simulink model "LKAS_AutoSave_DF_20220408_1006_SW62"  (R2018b)
settings: Solver=FixedStepDiscrete  StartTime=0.0  StopTime=10.0  FixedStep=0.01  RelTol=1e-3
undefined symbols (not defined in the file): LKA_CarWidth, LKA_SampleTime, LKA_StrRatio_C, LKA_Veh2CamL_C, LKA_Veh2CamW_C, LKA_WhlBaseL_C, LL_CompHdAg_C, LL_CompSWA_C, LL_CrvtPrvwT_C, LL_DesDvt_C, LL_DvtComp_C, LL_DvtPrvwT_C, LL_DvtSpdDet_vDvtSpdMin_C, LL_HandsOff_ExitTime, LL_HandsOff_TextTime, LL_HandsOff_WarnTime, LL_HdAgExT_C, LL_HdAgPrvwT_C, LL_LAccMax_C, LL_LAccRMax_C, LL_LDW_EarliestWarnLine_C, LL_LDW_LatestWarnLine_C, LL_LDWS_SUPPRESS_HEADING, LL_LFClb_TFC_FfCtlRatio_C, LL_LFClb_TFC_KdBalance_C, LL_LFClb_TFC_KdMaxSWA_C, LL_LFClb_TFC_KdV1_C, LL_LFClb_TFC_KdV2_C, LL_LFClb_TFC_KdVehSpdLwr_C, LL_LFClb_TFC_KdVehSpdUpr_C, LL_LFClb_TFC_Ki_C, LL_LFClb_TFC_KiMaxSWA_C, LL_LFClb_TFC_Kp_C, LL_LFClb_TFC_KpKlat_C, LL_LFClb_TFC_KpV1_C, LL_LFClb_TFC_KpV2_C, LL_LFClb_TFC_KpVehSpdLwr_C, LL_LFClb_TFC_KpVehSpdUpr_C, LL_LFClb_TFC_PrvwT_C, LL_LKA_EarliestWarnLine_C, LL_LKA_LatestWarnLine_C, LL_LKAExPrcs_ExitC0Dvt, LL_LKAExPrcs_ExitC0Swt, LL_LKAExPrcs_tiExitDelayTime3, LL_LKAExPrcs_tiExitTime1, LL_LKAExPrcs_tiExitTime2, LL_LKAExPrcs_tiExitTime3, LL_LKAS_OUT_OF_CONTROL_LAT_VEL, LL_LKAS_OUT_OF_CONTROL_TTLC, LL_LKASWASyn_M0, LL_LKASWASyn_M1, LL_LKASWASyn_M2, LL_LKASWASyn_M3D, LL_LKASWASyn_M3K_DT, LL_LKASWASyn_M3K_MSD, LL_LKASWASyn_M4K, LL_LKASWASyn_SWAaddMax, LL_LKASWASyn_T2, LL_LKASWASyn_tiTrqSwaRtTime, LL_LKASWASyn_tiTrqSwaTime ... (+47)
libraries: simulink x234, canmsglib x6, dspstat3 x3, simulink_extras x1
(part 3 of 16)

== system LKAS_AutoSave_DF_20220408_1006_SW62/LKAS/Output ==
  bsLLOut : Inport
  Bus Selector : BusSelector  OutputSignals=Vehicle_Lane_Display,LDW_Status_Display,LKA_Status_Display,LDW_Flag,Hands_Off_Warning,HapticAlarmReq,LKA_Action_Indication,HMI_Popup_Status,LKA_Torque_Req,LKA_TorqueReq_Value,EPS_State_Ctl,LKA_SWA_Control,EPS_Factor_Control,EPS_LKA_Control
  Cast To Single{1..9,12,14..16} (13 alike) : DataTypeConversion  OutDataTypeStr=UInt8
  Cast To Single10 : DataTypeConversion  OutDataTypeStr=T_M_Nm_Float32
  Cast To Single11 : DataTypeConversion  OutDataTypeStr=T_M_Nm_Float32
  Cast To Single13 : DataTypeConversion  OutDataTypeStr=T_M_Nm_Float32
  Ground : Ground
  Ground1 : Ground
  Vehicle_Lane_Display : Outport
  LDW_Status_Display : Outport  Port=2
  LKA_Status_Display : Outport  Port=3
  ELK_Status_Display : Outport  Port=4
  LDW_Flag : Outport  Port=5
  Hands_Off_Warning : Outport  Port=6
  HapticAlarmReq : Outport  Port=7
  LKA_Action_Indication : Outport  Port=8
  HMI_Popup_Status : Outport  Port=9
  HMI_ELKPopupMessage : Outport  Port=10
  LKA_TorqueReq : Outport  Port=11
  LKA_TorqueReq_Value : Outport  Port=12
  EPS_State_Control : Outport  Port=13
  LKA_SWA_Control : Outport  Port=14
  EPS_Factor_Control : Outport  Port=15
  EPS_LKA_Control : Outport  Port=16
  wires:
  Ground1/1 -> Cast To Single16/1  "<HMI_ELKPopupMessage>"
  Bus Selector/6 -> Cast To Single15/1  "<HapticAlarmReq>"
  Ground/1 -> Cast To Single14/1  "<ELK_Status_Display>"
  Cast To Single16/1 -> HMI_ELKPopupMessage/1  "HMI_ELKPopupMessage"
  Cast To Single14/1 -> ELK_Status_Display/1  "ELK_Status_Display"
  Cast To Single15/1 -> HapticAlarmReq/1  "HapticAlarmReq"
  Bus Selector/2 -> Cast To Single2/1  "<LDW_Status_Display>"
  Bus Selector/14 -> Cast To Single9/1  "<EPS_LKA_Control>"
  Bus Selector/12 -> Cast To Single11/1  "<LKA_SWA_Control>"
  bsLLOut/1 -> Bus Selector/1  "bsLLOutput"
  Bus Selector/11 -> Cast To Single8/1  "<EPS_State_Ctl>"
  Bus Selector/1 -> Cast To Single1/1  "<Vehicle_Lane_Display>"
  Bus Selector/5 -> Cast To Single5/1  "<Hands_Off_Warning>"
  Bus Selector/8 -> Cast To Single7/1  "<HMI_Popup_Status>"
  Bus Selector/7 -> Cast To Single6/1  "<LKA_Action_Indication>"
  Bus Selector/13 -> Cast To Single10/1  "<EPS_Factor_Control>"
  Bus Selector/3 -> Cast To Single3/1  "<LKA_Status_Display>"
  Bus Selector/4 -> Cast To Single4/1  "<LDW_Flag>"
  Bus Selector/9 -> Cast To Single12/1  "<LKA_Torque_Req>"
  Bus Selector/10 -> Cast To Single13/1  "<LKA_TorqueReq_Value>"
  Cast To Single13/1 -> LKA_TorqueReq_Value/1  "LKA_TorqueReq_Value"
  Cast To Single12/1 -> LKA_TorqueReq/1  "LKA_TorqueReq"
  Cast To Single11/1 -> LKA_SWA_Control/1  "LKA_SWA_Control"
  Cast To Single10/1 -> EPS_Factor_Control/1  "EPS_Factor_Control"
  Cast To Single9/1 -> EPS_LKA_Control/1  "EPS_LKA_Control"
  Cast To Single8/1 -> EPS_State_Control/1  "EPS_State_Control"
  Cast To Single7/1 -> HMI_Popup_Status/1  "HMI_Popup_Status"
  Cast To Single6/1 -> LKA_Action_Indication/1  "LKA_Action_Indication"
  Cast To Single5/1 -> Hands_Off_Warning/1  "Hands_Off_Warning"
  Cast To Single4/1 -> LDW_Flag/1  "LDW_Flag"
  Cast To Single3/1 -> LKA_Status_Display/1  "LKA_Status_Display"
  Cast To Single2/1 -> LDW_Status_Display/1  "LDW_Status_Display"
  Cast To Single1/1 -> Vehicle_Lane_Display/1  "Vehicle_Lane_Display"

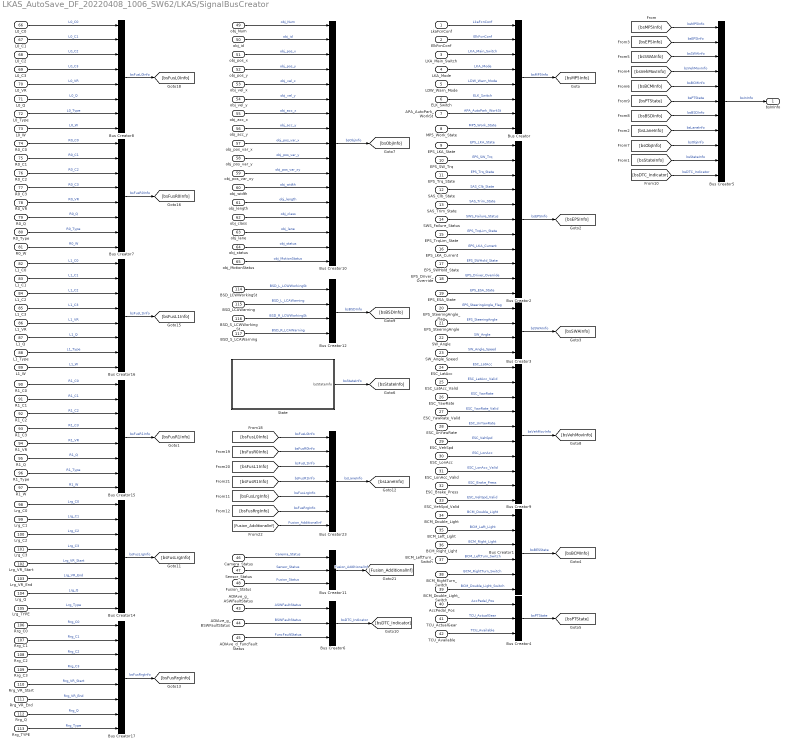
== system LKAS_AutoSave_DF_20220408_1006_SW62/LKAS/SignalBusCreator ==
  LkaFcnConf : Inport
  ElkFcnConf : Inport  Port=2
  LKA_Main_Switch : Inport  Port=3
  LKA_Mode : Inport  Port=4
  LDW_Warn_Mode : Inport  Port=5
  ELK_Switch : Inport  Port=6
  APA_AutoPark_WorkSt : Inport  Port=7
  MP5_Work_State : Inport  Port=8
  EPS_LKA_State : Inport  Port=9
  EPS_SW_Trq : Inport  Port=10
  EPS_Trq_State : Inport  Port=11
  SAS_Clb_State : Inport  Port=12
  SAS_Trim_State : Inport  Port=13
  SWS_Failure_Status : Inport  Port=14
  EPS_TrqLim_State : Inport  Port=15
  EPS_LKA_Current : Inport  Port=16
  EPS_SWHold_State : Inport  Port=17
  EPS_Driver_Override : Inport  Port=18
  EPS_ESA_State : Inport  Port=19
  EPS_SteeringAngle_Flag : Inport  Port=20
  EPS_SteeringAngle : Inport  Port=21
  SW_Angle : Inport  Port=22
  SW_Angle_Speed : Inport  Port=23
  ESC_LatAcc : Inport  Port=24
  ESC_LatAcc_Valid : Inport  Port=25
  ESC_YawRate : Inport  Port=26
  ESC_YawRate_Valid : Inport  Port=27
  ESC_UnYawRate : Inport  Port=28
  ESC_VehSpd : Inport  Port=29
  ESC_LonAcc : Inport  Port=30
  ESC_LonAcc_Valid : Inport  Port=31
  ESC_Brake_Press : Inport  Port=32
  ESC_VehSpd_Valid : Inport  Port=33
  BCM_Double_Light : Inport  Port=34
  BCM_Left_Light : Inport  Port=35
  BCM_Right_Light : Inport  Port=36
  BCM_LeftTurn_Switch : Inport  Port=37
  BCM_RightTurn_Switch : Inport  Port=38
  BCM_Double_Light_Switch : Inport  Port=39
  AccPedal_Pos : Inport  Port=40
  TCU_ActualGear : Inport  Port=41
  TCU_Available : Inport  Port=42
  ADIAve_g_ASWFaultStatus : Inport  Port=43
  ADIAve_g_BSWFaultStatus : Inport  Port=44
  ADIAve_d_FuncFaultStatus : Inport  Port=45
  Camera_Status : Inport  Port=46
  Sensor_Status : Inport  Port=47
  Fusion_Status : Inport  Port=48
  obj_Num : Inport  Port=49
  obj_id : Inport  Port=50
  obj_pos_x : Inport  Port=51
  obj_pos_y : Inport  Port=52
  obj_vel_x : Inport  Port=53
  obj_vel_y : Inport  Port=54
  obj_acc_x : Inport  Port=55
  obj_acc_y : Inport  Port=56
  obj_pos_var_x : Inport  Port=57
  obj_pos_var_y : Inport  Port=58
  obj_pos_var_xy : Inport  Port=59
  obj_width : Inport  Port=60
  obj_length : Inport  Port=61
  obj_class : Inport  Port=62
  obj_lane : Inport  Port=63
  obj_status : Inport  Port=64
  obj_MotionStatus : Inport  Port=65
  L0_C0 : Inport  Port=66
  L0_C1 : Inport  Port=67
  L0_C2 : Inport  Port=68
  L0_C3 : Inport  Port=69
  L0_VR : Inport  Port=70
  L0_Q : Inport  Port=71
  L0_Type : Inport  Port=72
  L0_W : Inport  Port=73
  R0_C0 : Inport  Port=74
  R0_C1 : Inport  Port=75
  R0_C2 : Inport  Port=76
  R0_C3 : Inport  Port=77
  R0_VR : Inport  Port=78
  R0_Q : Inport  Port=79
  R0_Type : Inport  Port=80
  R0_W : Inport  Port=81
  L1_C0 : Inport  Port=82
  L1_C1 : Inport  Port=83
  L1_C2 : Inport  Port=84
  L1_C3 : Inport  Port=85
  L1_VR : Inport  Port=86
  L1_Q : Inport  Port=87
  L1_Type : Inport  Port=88
  L1_W : Inport  Port=89
  R1_C0 : Inport  Port=90
  R1_C1 : Inport  Port=91
  R1_C2 : Inport  Port=92
  R1_C3 : Inport  Port=93
  R1_VR : Inport  Port=94
  R1_Q : Inport  Port=95
  R1_Type : Inport  Port=96
  R1_W : Inport  Port=97
  Lrg_C0 : Inport  Port=98
  Lrg_C1 : Inport  Port=99
  Lrg_C2 : Inport  Port=100
  Lrg_C3 : Inport  Port=101
  Lrg_VR_Start : Inport  Port=102
  Lrg_VR_End : Inport  Port=103
  Lrg_Q : Inport  Port=104
  Lrg_TYPE : Inport  Port=105
  Rrg_C0 : Inport  Port=106
  Rrg_C1 : Inport  Port=107
  Rrg_C2 : Inport  Port=108
  Rrg_C3 : Inport  Port=109
  Rrg_VR_Start : Inport  Port=110
  Rrg_VR_End : Inport  Port=111
  Rrg_Q : Inport  Port=112
  Rrg_TYPE : Inport  Port=113
  BSD_LCWWorkingSt : Inport  Port=114
  BSD_LCAWarning : Inport  Port=115
  BSD_S_LCWWorkingSt : Inport  Port=116
  BSD_S_LCAWarning : Inport  Port=117
  Bus Creator{,7..8,14..17} (7 alike) : BusCreator  Inputs=8
  Bus Creator1 : BusCreator  Inputs=6
  Bus Creator10 : BusCreator  Inputs=17
  Bus Creator11 : BusCreator  Inputs=3
  Bus Creator12 : BusCreator  Inputs=4
  Bus Creator2 : BusCreator  Inputs=11
  Bus Creator23 : BusCreator  Inputs=7
  Bus Creator3 : BusCreator  Inputs=4
  Bus Creator4 : BusCreator  Inputs=3
  Bus Creator5 : BusCreator  Inputs=11
  Bus Creator6 : BusCreator  Inputs=3
  Bus Creator9 : BusCreator  Inputs=10
  State : Subsystem
  bsInInfo : Outport
  wires:
  [bsFusRrgInfo] -> Bus Creator23/6  "bsFusRrgInfo"
  [bsFusLrgInfo] -> Bus Creator23/5  "bsFusLrgInfo"
  Rrg_TYPE/1 -> Bus Creator17/8  "Rrg_Type"
  Rrg_Q/1 -> Bus Creator17/7  "Rrg_Q"
  Rrg_VR_End/1 -> Bus Creator17/6  "Rrg_VR_End"
  Rrg_VR_Start/1 -> Bus Creator17/5  "Rrg_VR_Start"
  Rrg_C3/1 -> Bus Creator17/4  "Rrg_C3"
  Rrg_C2/1 -> Bus Creator17/3  "Rrg_C2"
  Rrg_C1/1 -> Bus Creator17/2  "Rrg_C1"
  Rrg_C0/1 -> Bus Creator17/1  "Rrg_C0"
  Bus Creator17/1 -> [bsFusRrgInfo]  "bsFusRrgInfo"
  Bus Creator14/1 -> [bsFusLrgInfo]  "bsFusLrgInfo"
  Lrg_TYPE/1 -> Bus Creator14/8  "Lrg_Type"
  Lrg_Q/1 -> Bus Creator14/7  "Lrg_Q"
  Lrg_VR_End/1 -> Bus Creator14/6  "Lrg_VR_End"
  Lrg_VR_Start/1 -> Bus Creator14/5  "Lrg_VR_Start"
  Lrg_C3/1 -> Bus Creator14/4  "Lrg_C3"
  Lrg_C2/1 -> Bus Creator14/3  "Lrg_C2"
  Lrg_C1/1 -> Bus Creator14/2  "Lrg_C1"
  Lrg_C0/1 -> Bus Creator14/1  "Lrg_C0"
  [bsBSDInfo] -> Bus Creator5/7  "bsBSDInfo"
  Bus Creator12/1 -> [bsBSDInfo]  "bsBSDInfo"
  BSD_S_LCAWarning/1 -> Bus Creator12/4  "BSD_R_LCAWarning"
  BSD_S_LCWWorkingSt/1 -> Bus Creator12/3  "BSD_R_LCWWorkingSt"
  BSD_LCAWarning/1 -> Bus Creator12/2  "BSD_L_LCAWarning"
  BSD_LCWWorkingSt/1 -> Bus Creator12/1  "BSD_L_LCWWorkingSt"
  [bsObjInfo] -> Bus Creator5/9  "bsObjInfo"
  Bus Creator10/1 -> [bsObjInfo]  "bsObjInfo"
  obj_MotionStatus/1 -> Bus Creator10/17  "obj_MotionStatus"
  obj_status/1 -> Bus Creator10/16  "obj_status"
  obj_lane/1 -> Bus Creator10/15  "obj_lane"
  obj_class/1 -> Bus Creator10/14  "obj_class"
  obj_length/1 -> Bus Creator10/13  "obj_length"
  obj_width/1 -> Bus Creator10/12  "obj_width"
  obj_pos_var_xy/1 -> Bus Creator10/11  "obj_pos_var_xy"
  obj_pos_var_y/1 -> Bus Creator10/10  "obj_pos_var_y"
  obj_pos_var_x/1 -> Bus Creator10/9  "obj_pos_var_x"
  obj_acc_y/1 -> Bus Creator10/8  "obj_acc_y"
  obj_acc_x/1 -> Bus Creator10/7  "obj_acc_x"
  obj_vel_y/1 -> Bus Creator10/6  "obj_vel_y"
  obj_vel_x/1 -> Bus Creator10/5  "obj_vel_x"
  obj_pos_y/1 -> Bus Creator10/4  "obj_pos_y"
  obj_pos_x/1 -> Bus Creator10/3  "obj_pos_x"
  obj_id/1 -> Bus Creator10/2  "obj_id"
  obj_Num/1 -> Bus Creator10/1  "obj_Num"
  ELK_Switch/1 -> Bus Creator/6  "ELK_Switch"
  ElkFcnConf/1 -> Bus Creator/2  "ElkFcnConf"
  BCM_Double_Light_Switch/1 -> Bus Creator1/6  "BCM_Double_Light_Switch"
  ADIAve_d_FuncFaultStatus/1 -> Bus Creator6/3  "FuncFaultStatus"
  ADIAve_g_BSWFaultStatus/1 -> Bus Creator6/2  "BSWFaultStatus"
  ADIAve_g_ASWFaultStatus/1 -> Bus Creator6/1  "ASWFaultStatus"
  EPS_ESA_State/1 -> Bus Creator2/11  "EPS_ESA_State"
  LkaFcnConf/1 -> Bus Creator/1  "LkaFcnConf"
  LDW_Warn_Mode/1 -> Bus Creator/5  "LDW_Warn_Mode"
  APA_AutoPark_WorkSt/1 -> Bus Creator/7  "APA_AutoPark_WorkSt"
  MP5_Work_State/1 -> Bus Creator/8  "MP5_Work_State"
  Fusion_Status/1 -> Bus Creator11/3  "Fusion_Status"
  Sensor_Status/1 -> Bus Creator11/2  "Sensor_Status"
  Camera_Status/1 -> Bus Creator11/1  "Carema_Status"
  Bus Creator11/1 -> [Fusion_AdditionalInf]  "Fusion_AdditionalInf"
  EPS_Driver_Override/1 -> Bus Creator2/10  "EPS_Driver_Override"
  EPS_SteeringAngle/1 -> Bus Creator3/2  "EPS_SteeringAngle"
  EPS_SteeringAngle_Flag/1 -> Bus Creator3/1  "EPS_SteeringAngle_Flag"
  BCM_RightTurn_Switch/1 -> Bus Creator1/5  "BCM_RightTurn_Switch"
  BCM_LeftTurn_Switch/1 -> Bus Creator1/4  "BCM_LeftTurn_Switch"
  TCU_Available/1 -> Bus Creator4/3  "TCU_Available"
  R1_W/1 -> Bus Creator15/8  "R1_W"
  R1_Type/1 -> Bus Creator15/7  "R1_Type"
  R1_Q/1 -> Bus Creator15/6  "R1_Q"
  R1_VR/1 -> Bus Creator15/5  "R1_VR"
  R1_C3/1 -> Bus Creator15/4  "R1_C3"
  R1_C2/1 -> Bus Creator15/3  "R1_C2"
  R1_C1/1 -> Bus Creator15/2  "R1_C1"
  R1_C0/1 -> Bus Creator15/1  "R1_C0"
  L1_W/1 -> Bus Creator16/8  "L1_W"
  L1_Type/1 -> Bus Creator16/7  "L1_Type"
  L1_Q/1 -> Bus Creator16/6  "L1_Q"
  L1_VR/1 -> Bus Creator16/5  "L1_VR"
  L1_C3/1 -> Bus Creator16/4  "L1_C3"
  L1_C2/1 -> Bus Creator16/3  "L1_C2"
  L1_C1/1 -> Bus Creator16/2  "L1_C1"
  L1_C0/1 -> Bus Creator16/1  "L1_C0"
  R0_W/1 -> Bus Creator7/8  "R0_W"
  R0_Type/1 -> Bus Creator7/7  "R0_Type"
  R0_Q/1 -> Bus Creator7/6  "R0_Q"
  R0_VR/1 -> Bus Creator7/5  "R0_VR"
  R0_C3/1 -> Bus Creator7/4  "R0_C3"
  R0_C2/1 -> Bus Creator7/3  "R0_C2"
  R0_C1/1 -> Bus Creator7/2  "R0_C1"
  R0_C0/1 -> Bus Creator7/1  "R0_C0"
  L0_W/1 -> Bus Creator8/8  "L0_W"
  L0_Type/1 -> Bus Creator8/7  "L0_Type"
  L0_Q/1 -> Bus Creator8/6  "L0_Q"
  L0_VR/1 -> Bus Creator8/5  "L0_VR"
  L0_C3/1 -> Bus Creator8/4  "L0_C3"
  L0_C2/1 -> Bus Creator8/3  "L0_C2"
  L0_C1/1 -> Bus Creator8/2  "L0_C1"
  L0_C0/1 -> Bus Creator8/1  "L0_C0"
  LKA_Mode/1 -> Bus Creator/4  "LKA_Mode"
  LKA_Main_Switch/1 -> Bus Creator/3  "LKA_Main_Switch"
  EPS_SWHold_State/1 -> Bus Creator2/9  "EPS_SWHold_State"
  EPS_LKA_Current/1 -> Bus Creator2/8  "EPS_LKA_Current"
  EPS_TrqLim_State/1 -> Bus Creator2/7  "EPS_TrqLim_State"
  SAS_Trim_State/1 -> Bus Creator2/5  "SAS_Trim_State"
  SAS_Clb_State/1 -> Bus Creator2/4  "SAS_Clb_State"
  EPS_Trq_State/1 -> Bus Creator2/3  "EPS_Trq_State"
  EPS_SW_Trq/1 -> Bus Creator2/2  "EPS_SW_Trq"
  EPS_LKA_State/1 -> Bus Creator2/1  "EPS_LKA_State"
  ESC_VehSpd_Valid/1 -> Bus Creator9/10  "ESC_VehSpd_Valid"
  ESC_Brake_Press/1 -> Bus Creator9/9  "ESC_Brake_Press"
  ESC_LonAcc_Valid/1 -> Bus Creator9/8  "ESC_LonAcc_Valid"
  ESC_LonAcc/1 -> Bus Creator9/7  "ESC_LonAcc"
  ESC_VehSpd/1 -> Bus Creator9/6  "ESC_VehSpd"
  ESC_UnYawRate/1 -> Bus Creator9/5  "ESC_UnYawRate"
  ESC_YawRate_Valid/1 -> Bus Creator9/4  "ESC_YawRate_Valid"
  ESC_YawRate/1 -> Bus Creator9/3  "ESC_YawRate"
  ESC_LatAcc_Valid/1 -> Bus Creator9/2  "ESC_LatAcc_Valid"
  ESC_LatAcc/1 -> Bus Creator9/1  "ESC_LatAcc"
  SWS_Failure_Status/1 -> Bus Creator2/6  "SWS_Failure_Status"
  SW_Angle_Speed/1 -> Bus Creator3/4  "SW_Angle_Speed"
  SW_Angle/1 -> Bus Creator3/3  "SW_Angle"
  BCM_Right_Light/1 -> Bus Creator1/3  "BCM_Right_Light"
  BCM_Left_Light/1 -> Bus Creator1/2  "BCM_Left_Light"
  BCM_Double_Light/1 -> Bus Creator1/1  "BCM_Double_Light"
  TCU_ActualGear/1 -> Bus Creator4/2  "TCU_ActualGear"
  AccPedal_Pos/1 -> Bus Creator4/1  "AccPedal_Pos"
  Bus Creator5/1 -> bsInInfo/1  "bsInInfo"
  State/1(bsStateInfo) -> [bsStateInfo]  "bsStateInfo"
  Bus Creator6/1 -> [bsDTC_Indicator]  "bsDTC_Indicator"
  [Fusion_AdditionalInf] -> Bus Creator23/7  "Fusion_AdditionalInf"
  Bus Creator23/1 -> [bsLaneInfo]  "bsLaneInfo"
  [bsFusR1Info] -> Bus Creator23/4  "bsFusR1Info"
  [bsFusL1Info] -> Bus Creator23/3  "bsFusL1Info"
  [bsFusR0Info] -> Bus Creator23/2  "bsFusR0Info"
  [bsFusL0Info] -> Bus Creator23/1  "bsFusL0Info"
  Bus Creator8/1 -> [bsFusL0Info]  "bsFusL0Info"
  Bus Creator15/1 -> [bsFusR1Info]  "bsFusR1Info"
  Bus Creator16/1 -> [bsFusL1Info]  "bsFusL1Info"
  Bus Creator7/1 -> [bsFusR0Info]  "bsFusR0Info"
  Bus Creator4/1 -> [bsPTState]  "bsPTState"
  [bsDTC_Indicator] -> Bus Creator5/11  "bsDTC_Indicator"
  [bsStateInfo] -> Bus Creator5/10  "bsStateInfo"
  [bsMP5Info] -> Bus Creator5/1  "bsMP5Info"
  [bsPTState] -> Bus Creator5/6  "bsPTState"
  [bsBCMInfo] -> Bus Creator5/5  "bsBCMInfo"
  [bsSWAInfo] -> Bus Creator5/3  "bsSWAInfo"
  [bsVehMovInfo] -> Bus Creator5/4  "bsVehMovInfo"
  [bsEPSInfo] -> Bus Creator5/2  "bsEPSInfo"
  [bsLaneInfo] -> Bus Creator5/8  "bsLaneInfo"
  Bus Creator/1 -> [bsMP5Info]  "bsMP5Info"
  Bus Creator2/1 -> [bsEPSInfo]  "bsEPSInfo"
  Bus Creator1/1 -> [bsBCMInfo]  "bsBESState"
  Bus Creator3/1 -> [bsSWAInfo]  "bsSWAInfo"
  Bus Creator9/1 -> [bsVehMovInfo]  "bsVehMovInfo"

== system LKAS_AutoSave_DF_20220408_1006_SW62/LKAS/LL/Fault_Diagnostic ==
  bsInInfo : Inport
  ASWFaultStatus_Unpack : Subsystem
  BSWFaultStatus_Unpack : Subsystem
  Bus Creator : BusCreator  Inputs=3
  Bus Selector4 : BusSelector  OutputSignals=bsDTC_Indicator.ASWFaultStatus,bsDTC_Indicator.BSWFaultStatus,bsDTC_Indicator.FuncFaultStatus
  FuncFaultStatus_Unpack : Subsystem
  bsFaultStatus : Outport
  wires:
  Bus Creator/1 -> bsFaultStatus/1  "bsFaultStatus"
  FuncFaultStatus_Unpack/1(bsFuncFaultStatus) -> Bus Creator/3  "bsFuncFaultStatus"
  BSWFaultStatus_Unpack/1(bsBSWFaultStatus) -> Bus Creator/2  "bsBSWFaultStatus"
  ASWFaultStatus_Unpack/1(bsASWFaultStatus) -> Bus Creator/1  "bsASWFaultStatus"
  [FuncFaultStatus] -> FuncFaultStatus_Unpack/1(FuncFaultStatus)
  [BSWFaultStatus] -> BSWFaultStatus_Unpack/1(BSWFaultStatus), ASWFaultStatus_Unpack/2(BSWFaultStatus)
  [ASWFaultStatus] -> ASWFaultStatus_Unpack/1(ASWFaultStatus)
  Bus Selector4/3 -> [FuncFaultStatus]  "<FuncFaultStatus>"
  Bus Selector4/2 -> [BSWFaultStatus]  "<BSWFaultStatus>"
  Bus Selector4/1 -> [ASWFaultStatus]  "<ASWFaultStatus>"
  bsInInfo/1 -> Bus Selector4/1

== system LKAS_AutoSave_DF_20220408_1006_SW62/LKAS/LL/Human Machine Interface (HMI) ==
  HMI_bsInfo : Inport
  HMI_bsLLState : Inport  Port=2
  HMI_bsLDWWarnInfo : Inport  Port=3
  HMI_bsLLClb : Inport  Port=4
  Bus Creator2 : BusCreator  Inputs=8
  Bus Selector : BusSelector  OutputSignals=bsConstantClb.LKA_SampleTime,bsLLSMConClb.DisblCClb.LL_HandsOff_TextTime,bsLLSMConClb.DisblCClb.LL_HandsOff_WarnTime,bsLLSMConClb.DisblCClb.LL_RlsDet_tiTrqChkT_DISABLE,bsLLSMConClb.DisblCClb.LL_RlsDet_tiTrqChkT_EPS_DISABLE
  Bus Selector1 : BusSelector  OutputSignals=LKA_Mode,LKA_State,LDW_State
  Bus Selector5 : BusSelector  OutputSignals=bsLaneInfo.bsR0Info.R0_Q,bsLaneInfo.bsL0Info.L0_Q,bsLaneInfo.Fusion_AdditionalInf.Carema_Status,bsEPSInfo,bsMP5Info.LDW_Warn_Mode
  Cast To Single{,1..6,8} (8 alike) : DataTypeConversion  OutDataTypeStr=uint8
  HMI_Popup_Status : MATLAB Function  TreatAsAtomicUnit=on
  Hands_Off_Warning : MATLAB Function  TreatAsAtomicUnit=on
  HapticAlarmReq : MATLAB Function  TreatAsAtomicUnit=on
  LDW_Flag : MATLAB Function  TreatAsAtomicUnit=on
  LKA_action_indication : MATLAB Function  TreatAsAtomicUnit=on
  Status_Display : MATLAB Function  TreatAsAtomicUnit=on
  Subsystem : Subsystem
  Vehicle_Lane_Display : MATLAB Function  TreatAsAtomicUnit=on
  HMI_LDWLKA : Outport
  wires:
  Bus Selector/5 -> Subsystem/8(LL_RlsDet_tiTrqChkT_EPS_DISABLE)  "<LL_RlsDet_tiTrqChkT_EPS_DISABLE>"
  Bus Selector/4 -> Subsystem/7(LL_RlsDet_tiTrqChkT_DISABLE)  "<LL_RlsDet_tiTrqChkT_DISABLE>"
  [HMI_Popup_Status] -> Cast To Single6/1
  [LKA_Action_Indication] -> Cast To Single5/1
  [HapticAlarmReq] -> Cast To Single8/1
  [LDW_Flag] -> HapticAlarmReq/2(LDW_Flag)
  Bus Selector5/5 -> LDW_Flag/4(LDW_Warn_Mode), HapticAlarmReq/1(LDW_Warn_Mode)  "<LDW_Warn_Mode>"
  [LDW_Flag] -> Cast To Single3/1
  [Hands_Off_Warning] -> Cast To Single4/1
  [LKA_Status_Display] -> Cast To Single2/1
  [LDW_Status_Display] -> Cast To Single1/1
  [Vehicle_Lane_Display] -> Cast To Single/1
  HMI_bsLLState/1 -> Bus Selector1/1
  HMI_bsInfo/1 -> Bus Selector5/1
  HapticAlarmReq/1(HapticAlarmReq) -> [HapticAlarmReq]  "HapticAlarmReq"
  Cast To Single8/1 -> Bus Creator2/6  "HapticAlarmReq"
  Bus Selector/3 -> Subsystem/6(LL_HandsOff_WarnTime)  "<LL_HandsOff_WarnTime>"
  Bus Selector/2 -> Subsystem/5(LL_HandsOff_TextTime)  "<LL_HandsOff_TextTime>"
  Bus Selector/1 -> Subsystem/4(LKA_SampleTime)  "<LKA_SampleTime>"
  HMI_bsLLClb/1 -> Bus Selector/1  "HMI_bsLLClb"
  HMI_bsLDWWarnInfo/1 -> LDW_Flag/3(LDWWarnInfo)
  Subsystem/1(HandsOff2_Warn) -> Hands_Off_Warning/1(HandsOff)
  Subsystem/2(HandsOff1_Text) -> HMI_Popup_Status/2(HandsOff1_Text)
  Bus Selector5/4 -> Subsystem/3(bsEPSInfo)  "<bsEPSInfo>"
  Bus Selector5/1 -> Vehicle_Lane_Display/4(R0_Q)  "<R0_Q>"
  Bus Selector5/3 -> HMI_Popup_Status/3(Camera_Status)  "<Carema_Status>"
  Bus Selector1/1 -> LDW_Flag/1(LKA_Mode), Status_Display/1(LKA_Mode), Vehicle_Lane_Display/1(LKA_Mode), LKA_action_indication/1(LKA_Mode), HMI_Popup_Status/1(LKA_Mode)  "<LKA_Mode>"
  Bus Selector5/2 -> Vehicle_Lane_Display/5(L0_Q)  "<L0_Q>"
  Bus Selector1/3 -> Subsystem/1(LDW_State), Vehicle_Lane_Display/3(LDW_State), Status_Display/2(LDW_STATE)  "<LDW_State>"
  Bus Selector1/2 -> Vehicle_Lane_Display/2(LKA_State), Status_Display/3(LKA_STATE), LDW_Flag/2(LKA_State), LKA_action_indication/2(LKA_STATE), Subsystem/2(LKA_State)  "<LKA_State>"
  Cast To Single4/1 -> Bus Creator2/5  "Hands_Off_Warning"
  LKA_action_indication/1(LKA_Action_Indication) -> [LKA_Action_Indication]  "LKA_Action_Indication"
  Cast To Single6/1 -> Bus Creator2/8  "HMI_Popup_Status"
  Cast To Single/1 -> Bus Creator2/1  "Vehicle_Lane_Display"
  Vehicle_Lane_Display/1(Vehicle_Lane_Display) -> [Vehicle_Lane_Display]  "Vehicle_Lane_Display"
  Cast To Single3/1 -> Bus Creator2/4  "LDW_Flag"
  Status_Display/2(LKA_Status_Display) -> [LKA_Status_Display]  "LKA_Status_Display"
  Cast To Single1/1 -> Bus Creator2/2  "LDW_Status_Display"
  HMI_Popup_Status/1(HMI_Popup_Status) -> [HMI_Popup_Status]  "HMI_Popup_Status"
  Status_Display/1(LDW_Status_Display) -> [LDW_Status_Display]  "LDW_Status_Display"
  LDW_Flag/1(LDW_Flag) -> [LDW_Flag]  "LDW_Flag"
  Cast To Single2/1 -> Bus Creator2/3  "LKA_Status_Display"
  Cast To Single5/1 -> Bus Creator2/7  "LKA_Action_Indication"
  Hands_Off_Warning/1(Hands_Off_Warning) -> [Hands_Off_Warning]  "Hands_Off_Warning"
  Bus Creator2/1 -> HMI_LDWLKA/1

== system LKAS_AutoSave_DF_20220408_1006_SW62/LKAS/LL/LL Inputs Mapping ==
  bsInInfo : Inport
  bsLLClb : Inport  Port=2
  Bus Creator : BusCreator  Inputs=7
  Bus Selector : BusSelector  OutputSignals=bsMP5Info,bsLaneInfo,bsEPSInfo,bsVehMovInfo,bsSWAInfo,bsBCMInfo,bsPTState
  bsBCMInfo : Subsystem
  bsEPSInfo : Subsystem
  bsLaneInfo : Subsystem
  bsMP5Info : Subsystem
  bsPTState : Subsystem
  bsSWAInfo : Subsystem
  bsVehMovInfo : Subsystem
  bsInfo : Outport
  wires:
  bsLLClb/1 -> bsLaneInfo/1(bsLLClb)
  bsInInfo/1 -> Bus Selector/1
  Bus Creator/1 -> bsInfo/1
  Bus Selector/2 -> bsLaneInfo/2(bsLaneInfoIn)  "<bsLaneInfo>"
  Bus Selector/3 -> bsEPSInfo/1(bsEPSInfoIn)  "<bsEPSInfo>"
  bsEPSInfo/1(bsEPSInfoOut) -> Bus Creator/3  "bsEPSInfo"
  Bus Selector/4 -> bsVehMovInfo/1(bsVehMovInfoIn)  "<bsVehMovInfo>"
  bsVehMovInfo/1(bsVehMovInfoOut) -> Bus Creator/4  "bsVehMovInfo"
  Bus Selector/5 -> bsSWAInfo/1(bsSWAInfoIn)  "<bsSWAInfo>"
  Bus Selector/6 -> bsBCMInfo/1(bsBCMInfoIn)  "<bsBCMInfo>"
  Bus Selector/1 -> bsMP5Info/1(bsMP5InfoIn)  "<bsMP5Info>"
  bsMP5Info/1(bsMP5InfoOut) -> Bus Creator/1  "bsMP5Info"
  bsBCMInfo/1(bsBCMInfoOut) -> Bus Creator/6  "bsBCMInfo"
  Bus Selector/7 -> bsPTState/1(bsPTStateIn)  "<bsPTState>"
  bsPTState/1(bsPTStateOut) -> Bus Creator/7  "bsPTState"
  bsLaneInfo/1(bsLaneInfoOut) -> Bus Creator/2  "bsLaneInfo"
  bsSWAInfo/1(bsSWAInfoOut) -> Bus Creator/5  "bsSWAInfo"

== system LKAS_AutoSave_DF_20220408_1006_SW62/LKAS/LL/LLOn ==
  bsInInfo : Inport
  bsLLClb : Inport  Port=2
  bsSignalFault : Inport  Port=3
  Enable : EnablePort  StatesWhenEnabling=reset
      settings: AttributesFormatString=states = %<StatesWhenEnabling>
  LDW : Subsystem  Description=|  TreatAsAtomicUnit=on
      | Block Name: Lane Departure Warning
      | Ab.: LDW
      | No.: 1.3.0.0
      | Rev: 0.0.1
      | Update Date: 19-3-26
  LKA : Subsystem  Description=|  TreatAsAtomicUnit=on
      | Block Name: Lane Keeping Assistance
      | Ab.: LKA
      | No.: 1.2.0.0
      | Rev: 0.0.1
      | Update Date: 19-5-13
  LKA Input Processing (LKAInP) : Subsystem
  LL State Determination (LLStateDet) : Subsystem
  LL_Mon : Subsystem
  bsLLState : Outport  OutputWhenDisabled=reset  InitialOutput=0
      settings: AttributesFormatString=%<OutputWhenDisabled> = %<InitialOutput>
  LDW_Flag : Outport  Port=2  OutputWhenDisabled=reset  InitialOutput=0
      settings: AttributesFormatString=%<OutputWhenDisabled> = %<InitialOutput>
  phiSWACmd : Outport  Port=3  OutputWhenDisabled=reset  InitialOutput=0
      settings: AttributesFormatString=%<OutputWhenDisabled> = %<InitialOutput>
  M : Outport  Port=4  OutputWhenDisabled=reset  InitialOutput=0
      settings: AttributesFormatString=%<OutputWhenDisabled> = %<InitialOutput>
  LLMon : Outport  Port=5
      settings: AttributesFormatString=%<OutputWhenDisabled> = %<InitialOutput>
  wires:
  LL State Determination (LLStateDet)/5(Fault_Reason) -> LL_Mon/2(Fault_Reason)
  LL State Determination (LLStateDet)/4(Disable_Reason) -> LL_Mon/1(Disable_Reason)
  [ActFlg] -> LKA Input Processing (LKAInP)/3(ActFlg)
  [bsLLClb] -> LKA/3(bsLLClb)
  LL_Mon/1(LLMon) -> LLMon/1
  [LKAMon] -> LL_Mon/3(LKAMon)
  LKA/4(LKAMon) -> [LKAMon]
  LKA/3(LKA_M) -> M/1  "OutputM"
  bsSignalFault/1 -> LL State Determination (LLStateDet)/5(bsSignalFault)
  LKA/1(LKA_ExitFlg) -> [ExitFlg]
  LKA/2(LKA_phiSWACmd) -> phiSWACmd/1  "OutputSWACmd"
  [ExitFlg] -> LL State Determination (LLStateDet)/4(ExitFlg)
  bsInInfo/1 -> LKA Input Processing (LKAInP)/1(bsInInfo), LKA/1(bsInInfo), LL State Determination (LLStateDet)/1(bsInInfo)
  LDW/1(LDW_Flag) -> LDW_Flag/1  "LDW_Flag"
  LL State Determination (LLStateDet)/3(stLKAActvFlg) -> [ActFlg], LKA/Enable
  bsLLClb/1 -> [bsLLClb]
  LKA Input Processing (LKAInP)/1(bsLKAInPInfo) -> LDW/1(bsLKAInPInfo), LL State Determination (LLStateDet)/2(bsLKAInPInfo), LKA/2(bsLKAInPInfo)
  [bsLLClb] -> LDW/2(bsLLClb)
  LL State Determination (LLStateDet)/1(bsLLState) -> bsLLState/1
  [bsLLClb] -> LKA Input Processing (LKAInP)/2(bsLLClb)
  [bsLLClb] -> LL State Determination (LLStateDet)/3(bsLLClb)
  LL State Determination (LLStateDet)/2(stLDWActvFlg) -> LDW/Enable

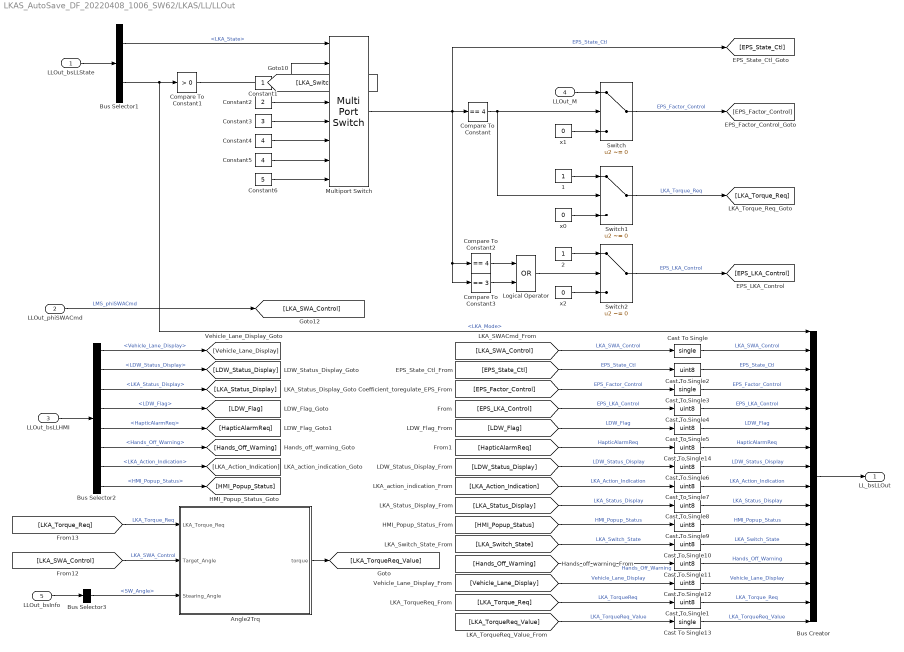
== system LKAS_AutoSave_DF_20220408_1006_SW62/LKAS/LL/LLOut ==
  LLOut_bsLLState : Inport
  LLOut_phiSWACmd : Inport  Port=2
  LLOut_bsLLHMI : Inport  Port=3
  LLOut_M : Inport  Port=4
  LLOut_bsInfo : Inport  Port=5
  1 : Constant  OutDataTypeStr=uint8
      settings: AttributesFormatString=DT: %<OutDataTypeStr>
  2 : Constant  OutDataTypeStr=uint8
      settings: AttributesFormatString=DT: %<OutDataTypeStr>
  Angle2Trq : Subsystem
  Bus Creator : BusCreator  Inputs=16
  Bus Selector1 : BusSelector  OutputSignals=LKA_State,LKA_Mode
  Bus Selector2 : BusSelector  OutputSignals=Vehicle_Lane_Display,LDW_Status_Display,LKA_Status_Display,LDW_Flag,HapticAlarmReq,Hands_Off_Warning,LKA_Action_Indication,HMI_Popup_Status
  Bus Selector3 : BusSelector  OutputSignals=bsSWAInfo.SW_Angle
  Cast To Single : DataTypeConversion  OutDataTypeStr=single
  Cast To Single{1..2,4..12,14} (12 alike) : DataTypeConversion  OutDataTypeStr=uint8
  Cast To Single13 : DataTypeConversion  OutDataTypeStr=single
  Cast To Single3 : DataTypeConversion  OutDataTypeStr=single
  Compare To Constant : simulink/Logic and Bit Operations/Compare To Constant  relop===  const=4  OutDataTypeStr=boolean
  Compare To Constant1 : simulink/Logic and Bit Operations/Compare To Constant  relop=>  const=0  OutDataTypeStr=boolean
  Compare To Constant2 : simulink/Logic and Bit Operations/Compare To Constant  relop===  const=4  OutDataTypeStr=boolean
  Compare To Constant3 : simulink/Logic and Bit Operations/Compare To Constant  relop===  const=3  OutDataTypeStr=boolean
  Constant1 : Constant  OutDataTypeStr=uint8
  Constant2 : Constant  Value=2  OutDataTypeStr=uint8
  Constant3 : Constant  Value=3  OutDataTypeStr=uint8
  Constant4 : Constant  Value=4  OutDataTypeStr=uint8
  Constant5 : Constant  Value=4  OutDataTypeStr=uint8
  Constant6 : Constant  Value=5  OutDataTypeStr=uint8
  Logical Operator : Logic  Operator=OR  AllPortsSameDT=off  OutDataTypeStr=boolean
  Multiport Switch : MultiPortSwitch  DataPortOrder=Zero-based contiguous  Inputs=7  zeroidx=on
  Switch : Switch  Criteria=u2 ~= 0
      settings: AttributesFormatString=%<Criteria>
  Switch1 : Switch  Criteria=u2 ~= 0
      settings: AttributesFormatString=%<Criteria>
  Switch2 : Switch  Criteria=u2 ~= 0
      settings: AttributesFormatString=%<Criteria>
  x0 : Constant  Value=0  OutDataTypeStr=uint8
      settings: AttributesFormatString=DT: %<OutDataTypeStr>
  x1 : Constant  Value=0  OutDataTypeStr=uint8
      settings: AttributesFormatString=DT: %<OutDataTypeStr>
  x2 : Constant  Value=0  OutDataTypeStr=uint8
      settings: AttributesFormatString=DT: %<OutDataTypeStr>
  LL_bsLLOut : Outport
      settings: AttributesFormatString=Disable Action: %<OutputWhenDisabled>
  wires:
  Cast To Single14/1 -> Bus Creator/7  "HapticAlarmReq"
  [HapticAlarmReq] -> Cast To Single14/1  "HapticAlarmReq"
  Bus Selector2/5 -> [HapticAlarmReq]  "<HapticAlarmReq>"
  x2/1 -> Switch2/3
  2/1 -> Switch2/1
  Switch2/1 -> [EPS_LKA_Control]  "EPS_LKA_Control"
  Logical Operator/1 -> Switch2/2
  Compare To Constant3/1 -> Logical Operator/2
  Compare To Constant2/1 -> Logical Operator/1
  x1/1 -> Switch/3
  Bus Selector3/1 -> Angle2Trq/3(Stearing_Angle)  "<SW_Angle>"
  LLOut_bsInfo/1 -> Bus Selector3/1
  Angle2Trq/1(torque) -> [LKA_TorqueReq_Value]
  [LKA_SWA_Control] -> Angle2Trq/2(Target_Angle)  "LKA_SWA_Control"
  [LKA_Torque_Req] -> Angle2Trq/1(LKA_Torque_Req)  "LKA_Torque_Req"
  LLOut_phiSWACmd/1 -> [LKA_SWA_Control]  "LMS_phiSWACmd"
  x0/1 -> Switch1/3
  1/1 -> Switch1/1
  Switch1/1 -> [LKA_Torque_Req]  "LKA_Torque_Req"
  Bus Selector2/1 -> [Vehicle_Lane_Display]  "<Vehicle_Lane_Display>"
  Bus Selector2/8 -> [HMI_Popup_Status]  "<HMI_Popup_Status>"
  Bus Selector2/3 -> [LKA_Status_Display]  "<LKA_Status_Display>"
  Bus Selector2/4 -> [LDW_Flag]  "<LDW_Flag>"
  LLOut_bsLLHMI/1 -> Bus Selector2/1
  Bus Selector2/2 -> [LDW_Status_Display]  "<LDW_Status_Display>"
  Bus Selector2/7 -> [LKA_Action_Indication]  "<LKA_Action_Indication>"
  Bus Selector2/6 -> [Hands_Off_Warning]  "<Hands_Off_Warning>"
  Constant1/1 -> Multiport Switch/3, Multiport Switch/2
  Constant5/1 -> Multiport Switch/7
  Cast To Single11/1 -> Bus Creator/13  "Hands_Off_Warning"
  LLOut_M/1 -> Switch/1
  Cast To Single9/1 -> Bus Creator/11  "HMI_Popup_Status"
  Constant4/1 -> Multiport Switch/6
  Compare To Constant1/1 -> [LKA_Switch_State]
  LLOut_bsLLState/1 -> Bus Selector1/1
  [EPS_State_Ctl] -> Cast To Single2/1  "EPS_State_Ctl"
  Cast To Single12/1 -> Bus Creator/14  "Vehicle_Lane_Display"
  Cast To Single6/1 -> Bus Creator/8  "LDW_Status_Display"
  Switch/1 -> [EPS_Factor_Control]  "EPS_Factor_Control"
  Multiport Switch/1 -> Compare To Constant/1, [EPS_State_Ctl], Compare To Constant3/1, Compare To Constant2/1  "EPS_State_Ctl"
  Constant3/1 -> Multiport Switch/5
  Cast To Single3/1 -> Bus Creator/4  "EPS_Factor_Control"
  Bus Creator/1 -> LL_bsLLOut/1
  Cast To Single2/1 -> Bus Creator/3  "EPS_State_Ctl"
  Constant2/1 -> Multiport Switch/4
  Bus Selector1/2 -> Compare To Constant1/1, Bus Creator/1  "<LKA_Mode>"
  Cast To Single10/1 -> Bus Creator/12  "LKA_Switch_State"
  Cast To Single4/1 -> Bus Creator/5  "EPS_LKA_Control"
  Cast To Single8/1 -> Bus Creator/10  "LKA_Status_Display"
  [Hands_Off_Warning] -> Cast To Single11/1  "Hands_Off_Warning"
  [LKA_Switch_State] -> Cast To Single10/1  "LKA_Switch_State"
  [LDW_Status_Display] -> Cast To Single6/1  "LDW_Status_Display"
  Cast To Single/1 -> Bus Creator/2  "LKA_SWA_Control"
  [LKA_SWA_Control] -> Cast To Single/1  "LKA_SWA_Control"
  [LKA_Status_Display] -> Cast To Single8/1  "LKA_Status_Display"
  Bus Selector1/1 -> Multiport Switch/1  "<LKA_State>"
  [HMI_Popup_Status] -> Cast To Single9/1  "HMI_Popup_Status"
  Cast To Single5/1 -> Bus Creator/6  "LDW_Flag"
  Constant6/1 -> Multiport Switch/8
  [LKA_Action_Indication] -> Cast To Single7/1  "LKA_Action_Indication"
  [EPS_Factor_Control] -> Cast To Single3/1  "EPS_Factor_Control"
  [LDW_Flag] -> Cast To Single5/1  "LDW_Flag"
  [EPS_LKA_Control] -> Cast To Single4/1  "EPS_LKA_Control"
  [Vehicle_Lane_Display] -> Cast To Single12/1  "Vehicle_Lane_Display"
  Compare To Constant/1 -> Switch1/2, Switch/2
  Cast To Single7/1 -> Bus Creator/9  "LKA_Action_Indication"
  [LKA_Torque_Req] -> Cast To Single1/1  "LKA_TorqueReq"
  Cast To Single1/1 -> Bus Creator/15  "LKA_Torque_Req"
  [LKA_TorqueReq_Value] -> Cast To Single13/1  "LKA_TorqueReq_Value"
  Cast To Single13/1 -> Bus Creator/16  "LKA_TorqueReq_Value"

== system LKAS_AutoSave_DF_20220408_1006_SW62/LKAS/LLClb/ConstantClb ==
  Bus Creator : BusCreator  Inputs=6
  Data Type Conversion{2..4,6,13,22} (6 alike) : DataTypeConversion  OutDataTypeStr=single
  LKA_CarWidth=1.8 : Constant  Value=LKA_CarWidth
  LKA_SampleTime=0.01 : Constant  Value=LKA_SampleTime  OutDataTypeStr=single
  LKA_StrRatio_C=15.3 : Constant  Value=LKA_StrRatio_C
  LKA_Veh2CamL_C=1.56 : Constant  Value=LKA_Veh2CamL_C
  LKA_Veh2CamW_C=0.9 : Constant  Value=LKA_Veh2CamW_C  OutDataTypeStr=single
  LKA_WhlBaseL_C=2.65 : Constant  Value=LKA_WhlBaseL_C
  Switch{,1..3,11,19} (6 alike) : Switch  Criteria=u2 ~= 0  OutDataTypeStr=single
  ConstantClb : Outport
  wires:
  LKA_Veh2CamW_C=0.9/1 -> Switch/3  "LKA_Veh2CamW_C"
  Data Type Conversion13/1 -> Switch/1, Switch/2
  Data Type Conversion2/1 -> Switch1/1, Switch1/2
  LKA_Veh2CamL_C=1.56/1 -> Switch1/3  "LKA_Veh2CamL_C"
  LKA_WhlBaseL_C=2.65/1 -> Switch2/3  "LKA_WhlBaseL_C"
  Data Type Conversion4/1 -> Switch2/1, Switch2/2
  Data Type Conversion6/1 -> Switch3/1, Switch3/2
  LKA_StrRatio_C=15.3/1 -> Switch3/3  "LKA_StrRatio_C"
  Data Type Conversion22/1 -> Switch11/1, Switch11/2
  LKA_CarWidth=1.8/1 -> Switch11/3  "LKA_CarWidth"
  Bus Creator/1 -> ConstantClb/1
  Switch3/1 -> Bus Creator/5  "LKA_StrRatio_C"
  Switch11/1 -> Bus Creator/6  "LKA_CarWidth"
  Switch1/1 -> Bus Creator/3  "LKA_Veh2CamL_C"
  Switch/1 -> Bus Creator/2  "LKA_Veh2CamW_C"
  Switch2/1 -> Bus Creator/4  "LKA_WhlBaseL_C"
  Switch19/1 -> Bus Creator/1  "LKA_SampleTime"
  Data Type Conversion3/1 -> Switch19/2, Switch19/1
  LKA_SampleTime=0.01/1 -> Switch19/3  "LKA_SampleTime"

== system LKAS_AutoSave_DF_20220408_1006_SW62/LKAS/LLClb/LDWClb ==
  Bus Creator : BusCreator  Inputs=1
  Data Type Conversion6 : DataTypeConversion  OutDataTypeStr=single
  LL_LDWS_SUPPRESS_HEADING=2 : Constant  Value=LL_LDWS_SUPPRESS_HEADING  OutDataTypeStr=single
  Switch2 : Switch  Criteria=u2 ~= 0  OutDataTypeStr=single
  LDWClb : Outport
  wires:
  Bus Creator/1 -> LDWClb/1
  Switch2/1 -> Bus Creator/1  "LL_LDWS_SUPPRESS_HEADING"
  LL_LDWS_SUPPRESS_HEADING=2/1 -> Switch2/3
  Data Type Conversion6/1 -> Switch2/1, Switch2/2

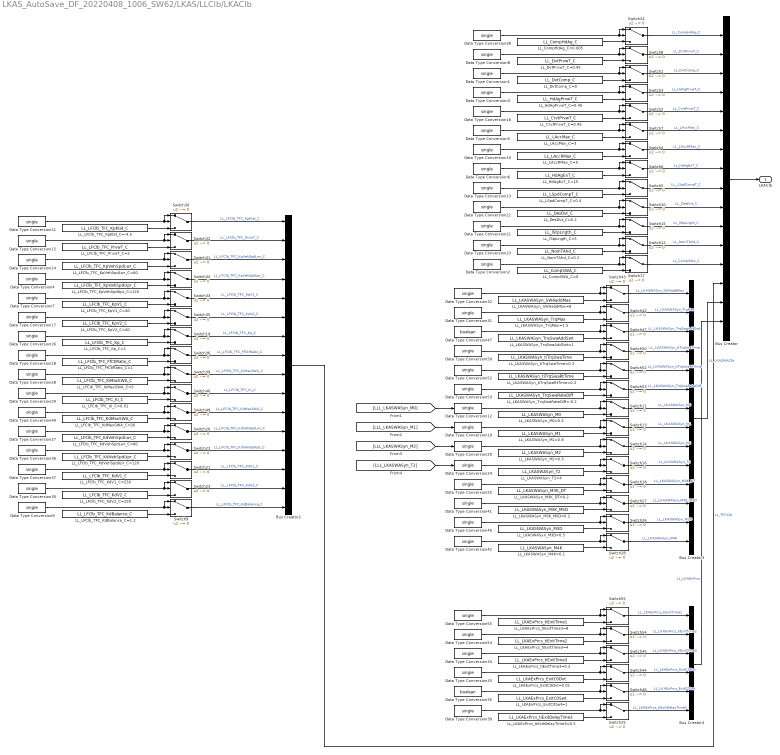
== system LKAS_AutoSave_DF_20220408_1006_SW62/LKAS/LLClb/LKAClb ==
  Bus Creator : BusCreator  Inputs=16
  Bus Creator2 : BusCreator  Inputs=16
  Bus Creator3 : BusCreator  Inputs=14
  Bus Creator4 : BusCreator  Inputs=6
  Data Type Conversion{1..34,36..42,49..50,52..55} (47 alike) : DataTypeConversion  OutDataTypeStr=single
  Data Type Conversion35 : DataTypeConversion  OutDataTypeStr=boolean
  Data Type Conversion47 : DataTypeConversion  OutDataTypeStr=boolean
  LL_CompHdAg_C=0.005 : Constant  Value=LL_CompHdAg_C  OutDataTypeStr=single
  LL_CompSWA_C=0 : Constant  Value=LL_CompSWA_C  OutDataTypeStr=single
  LL_CrvtPrvwT_C=0.45 : Constant  Value=LL_CrvtPrvwT_C  OutDataTypeStr=single
  LL_DesDvt_C=0.2 : Constant  Value=LL_DesDvt_C  OutDataTypeStr=single
  LL_DvtComp_C=0 : Constant  Value=LL_DvtComp_C  OutDataTypeStr=single
  LL_DvtPrvwT_C=0.45 : Constant  Value=LL_DvtPrvwT_C  OutDataTypeStr=single
  LL_HdAgExT_C=15 : Constant  Value=LL_HdAgExT_C  OutDataTypeStr=single
  LL_HdAgPrvwT_C=0.45 : Constant  Value=LL_HdAgPrvwT_C  OutDataTypeStr=single
  LL_LAccMax_C=3 : Constant  Value=LL_LAccMax_C  OutDataTypeStr=single
  LL_LAccRMax_C=5 : Constant  Value=LL_LAccRMax_C  OutDataTypeStr=single
  LL_LFClb_TFC_FfCtlRatio_C=1 : Constant  Value=LL_LFClb_TFC_FfCtlRatio_C  OutDataTypeStr=single
  LL_LFClb_TFC_KdBalance_C=1.2 : Constant  Value=LL_LFClb_TFC_KdBalance_C  OutDataTypeStr=single
  LL_LFClb_TFC_KdMaxSWA_C=20 : Constant  Value=LL_LFClb_TFC_KdMaxSWA_C  OutDataTypeStr=single
  LL_LFClb_TFC_KdV1_C=250 : Constant  Value=LL_LFClb_TFC_KdV1_C  OutDataTypeStr=single
  LL_LFClb_TFC_KdV2_C=250 : Constant  Value=LL_LFClb_TFC_KdV2_C  OutDataTypeStr=single
  LL_LFClb_TFC_KdVehSpdLwr_C=60 : Constant  Value=LL_LFClb_TFC_KdVehSpdLwr_C  OutDataTypeStr=single
  LL_LFClb_TFC_KdVehSpdUpr_C=120 : Constant  Value=LL_LFClb_TFC_KdVehSpdUpr_C  OutDataTypeStr=single
  LL_LFClb_TFC_KiMaxSWA_C=5 : Constant  Value=LL_LFClb_TFC_KiMaxSWA_C  OutDataTypeStr=single
  LL_LFClb_TFC_Ki_C=0.01 : Constant  Value=LL_LFClb_TFC_Ki_C  OutDataTypeStr=single
  LL_LFClb_TFC_KpKlat_C=-4.5 : Constant  Value=LL_LFClb_TFC_KpKlat_C  OutDataTypeStr=single
  LL_LFClb_TFC_KpV1_C=40 : Constant  Value=LL_LFClb_TFC_KpV1_C  OutDataTypeStr=single
  LL_LFClb_TFC_KpV2_C=40 : Constant  Value=LL_LFClb_TFC_KpV2_C  OutDataTypeStr=single
  LL_LFClb_TFC_KpVehSpdLwr_C=60 : Constant  Value=LL_LFClb_TFC_KpVehSpdLwr_C  OutDataTypeStr=single
  LL_LFClb_TFC_KpVehSpdUpr_C=120 : Constant  Value=LL_LFClb_TFC_KpVehSpdUpr_C  OutDataTypeStr=single
  LL_LFClb_TFC_Kp_C=1 : Constant  Value=LL_LFClb_TFC_Kp_C  OutDataTypeStr=single
  LL_LFClb_TFC_PrvwT_C=2 : Constant  Value=LL_LFClb_TFC_PrvwT_C  OutDataTypeStr=single
  LL_LKAExPrcs_ExitC0Dvt=0.01 : Constant  Value=LL_LKAExPrcs_ExitC0Dvt  OutDataTypeStr=single
  LL_LKAExPrcs_ExitC0Swt=1 : Constant  Value=LL_LKAExPrcs_ExitC0Swt  OutDataTypeStr=boolean
  LL_LKAExPrcs_tiExitDelayTime3=0.5 : Constant  Value=LL_LKAExPrcs_tiExitDelayTime3  OutDataTypeStr=single
  LL_LKAExPrcs_tiExitTime3=0.2 : Constant  Value=LL_LKAExPrcs_tiExitTime3  OutDataTypeStr=single
  LL_LKAExPrcs_tiExitTime3=4 : Constant  Value=LL_LKAExPrcs_tiExitTime2  OutDataTypeStr=single
  LL_LKAExPrcs_tiExitTime3=8 : Constant  Value=LL_LKAExPrcs_tiExitTime1  OutDataTypeStr=single
  LL_LKASWASyn_M0=0.4 : Constant  Value=LL_LKASWASyn_M0  OutDataTypeStr=single
  LL_LKASWASyn_M1=0.8 : Constant  Value=LL_LKASWASyn_M1  OutDataTypeStr=single
  LL_LKASWASyn_M2=0.3 : Constant  Value=LL_LKASWASyn_M2  OutDataTypeStr=single
  LL_LKASWASyn_M3D=0.5 : Constant  Value=LL_LKASWASyn_M3D  OutDataTypeStr=single
  LL_LKASWASyn_M3K_DT=0.2 : Constant  Value=LL_LKASWASyn_M3K_DT  OutDataTypeStr=single
  LL_LKASWASyn_M3K_MSD=0.2 : Constant  Value=LL_LKASWASyn_M3K_MSD  OutDataTypeStr=single
  LL_LKASWASyn_M4K=0.1 : Constant  Value=LL_LKASWASyn_M4K  OutDataTypeStr=single
  LL_LKASWASyn_SWAaddMax=8 : Constant  Value=LL_LKASWASyn_SWAaddMax  OutDataTypeStr=single
  LL_LKASWASyn_T2=4 : Constant  Value=LL_LKASWASyn_T2  OutDataTypeStr=single
  LL_LKASWASyn_TrqMax=1.5 : Constant  Value=LL_LKASWASyn_TrqMax  OutDataTypeStr=single
  LL_LKASWASyn_TrqSwaAddSwt=1 : Constant  Value=LL_LKASWASyn_TrqSwaAddSwt  OutDataTypeStr=boolean
  LL_LKASWASyn_TrqSwaRateDiff=-0.2 : Constant  Value=LL_LKASWASyn_TrqSwaRateDiff  OutDataTypeStr=single
  LL_LKASWASyn_tiTrqSwaRtTime=0.2 : Constant  Value=LL_LKASWASyn_tiTrqSwaRtTime  OutDataTypeStr=single
  LL_LKASWASyn_tiTrqSwaTime=0.3 : Constant  Value=LL_LKASWASyn_tiTrqSwaTime  OutDataTypeStr=single
  LL_LSpdCompT_C=0.4 : Constant  Value=LL_LSpdCompT_C  OutDataTypeStr=single
  LL_NomTAhd_C=0.2 : Constant  Value=LL_NomTAhd_C  OutDataTypeStr=single
  LL_lStpLngth_C=5 : Constant  Value=LL_lStpLngth_C  OutDataTypeStr=single
  Switch{1..28,30..36,39..40,42..45,49..50,52..55} (47 alike) : Switch  Criteria=u2 ~= 0  OutDataTypeStr=single
  Switch46 : Switch  Criteria=u2 ~= 0  OutDataTypeStr=boolean
  Switch47 : Switch  Criteria=u2 ~= 0  OutDataTypeStr=boolean
  LKAClb : Outport
  wires:
  Data Type Conversion42/1 -> Switch28/2, Switch28/1
  LL_LKASWASyn_M4K=0.1/1 -> Switch28/3
  Switch28/1 -> Bus Creator3/14  "LL_LKASWASyn_M4K"
  Switch27/1 -> Bus Creator3/12  "LL_LKASWASyn_M3K_MSD"
  LL_LKASWASyn_M3K_MSD=0.2/1 -> Switch27/3
  Data Type Conversion41/1 -> Switch27/1, Switch27/2
  Switch26/1 -> Bus Creator3/13  "LL_LKASWASyn_M3D"
  LL_LKASWASyn_M3D=0.5/1 -> Switch26/3
  Data Type Conversion40/1 -> Switch26/1, Switch26/2
  Data Type Conversion39/1 -> Switch25/2, Switch25/1
  Switch25/1 -> Bus Creator4/6  "LL_LKAExPrcs_tiExitDelayTime3"
  LL_LKAExPrcs_tiExitDelayTime3=0.5/1 -> Switch25/3
  LL_CompHdAg_C=0.005/1 -> Switch24/3
  Data Type Conversion38/1 -> Switch24/1, Switch24/2
  Switch24/1 -> Bus Creator/1  "LL_CompHdAg_C"
  Data Type Conversion37/1 -> Switch21/2, Switch21/1
  LL_LFClb_TFC_KdV2_C=250/1 -> Switch23/3
  Switch23/1 -> Bus Creator2/15  "LL_LFClb_TFC_KdV2_C"
  LL_LFClb_TFC_KdVehSpdUpr_C=120/1 -> Switch22/3
  Switch20/1 -> Bus Creator2/12  "LL_LFClb_TFC_KdVehSpdLwr_C"
  Switch22/1 -> Bus Creator2/13  "LL_LFClb_TFC_KdVehSpdUpr_C"
  Data Type Conversion27/1 -> Switch20/2, Switch20/1
  Data Type Conversion36/1 -> Switch22/2, Switch22/1
  LL_LFClb_TFC_KdV1_C=250/1 -> Switch21/3
  LL_LFClb_TFC_KdVehSpdLwr_C=60/1 -> Switch20/3
  Switch21/1 -> Bus Creator2/14  "LL_LFClb_TFC_KdV1_C"
  Data Type Conversion30/1 -> Switch23/2, Switch23/1
  LL_LFClb_TFC_Kp_C=1/1 -> Switch19/3
  Switch19/1 -> Bus Creator2/7  "LL_LFClb_TFC_Kp_C"
  Data Type Conversion26/1 -> Switch19/2, Switch19/1
  Bus Creator/1 -> LKAClb/1
  Switch8/1 -> Bus Creator/2  "LL_DvtPrvwT_C"
  Switch1/1 -> Bus Creator/3  "LL_DvtComp_C"
  Switch3/1 -> Bus Creator/4  "LL_HdAgPrvwT_C"
  Switch17/1 -> Bus Creator/13  "LL_CompSWA_C"
  Switch6/1 -> Bus Creator/8  "LL_HdAgExT_C"
  Switch7/1 -> Bus Creator/6  "LL_LAccMax_C"
  Switch4/1 -> Bus Creator/7  "LL_LAccRMax_C"
  Switch5/1 -> Bus Creator/9  "LL_LSpdCompT_C"
  Switch2/1 -> Bus Creator/5  "LL_CrvtPrvwT_C"
  Switch15/1 -> Bus Creator/11  "LL_lStpLngth_C"
  Switch10/1 -> Bus Creator/10  "LL_DesDvt_C"
  Switch12/1 -> Bus Creator/12  "LL_NomTAhd_C"
  LL_DvtPrvwT_C=0.45/1 -> Switch8/3
  Data Type Conversion8/1 -> Switch8/1, Switch8/2
  Data Type Conversion1/1 -> Switch1/2, Switch1/1
  LL_DvtComp_C=0/1 -> Switch1/3
  LL_CrvtPrvwT_C=0.45/1 -> Switch2/3
  Data Type Conversion16/1 -> Switch2/2, Switch2/1
  Data Type Conversion3/1 -> Switch3/2, Switch3/1
  LL_HdAgPrvwT_C=0.45/1 -> Switch3/3
  LL_HdAgExT_C=15/1 -> Switch6/3
  Data Type Conversion6/1 -> Switch6/2, Switch6/1
  Data Type Conversion13/1 -> Switch5/2, Switch5/1
  LL_LSpdCompT_C=0.4/1 -> Switch5/3
  LL_LAccRMax_C=5/1 -> Switch4/3
  Data Type Conversion10/1 -> Switch4/1, Switch4/2
  Data Type Conversion5/1 -> Switch7/2, Switch7/1
  LL_LAccMax_C=3/1 -> Switch7/3
  Data Type Conversion21/1 -> Switch15/2, Switch15/1
  Data Type Conversion23/1 -> Switch12/2, Switch12/1
  Data Type Conversion22/1 -> Switch10/2, Switch10/1
  Data Type Conversion2/1 -> Switch17/2, Switch17/1
  LL_DesDvt_C=0.2/1 -> Switch10/3
  LL_lStpLngth_C=5/1 -> Switch15/3
  LL_NomTAhd_C=0.2/1 -> Switch12/3
  LL_CompSWA_C=0/1 -> Switch17/3
  Bus Creator2/1 -> Bus Creator/14  "LL_TFCClb"
  Switch35/1 -> Bus Creator2/6  "LL_LFClb_TFC_KpV2_C"
  Switch30/1 -> Bus Creator2/1  "LL_LFClb_TFC_KpKlat_C"
  Switch31/1 -> Bus Creator2/3  "LL_LFClb_TFC_KpVehSpdLwr_C"
  Switch34/1 -> Bus Creator2/4  "LL_LFClb_TFC_KpVehSpdUpr_C"
  Switch33/1 -> Bus Creator2/5  "LL_LFClb_TFC_KpV1_C"
  Switch32/1 -> Bus Creator2/2  "LL_LFClb_TFC_PrvwT_C"
  LL_LFClb_TFC_KpV1_C=40/1 -> Switch33/3
  LL_LFClb_TFC_KpVehSpdLwr_C=60/1 -> Switch31/3
  LL_LFClb_TFC_PrvwT_C=2/1 -> Switch32/3
  Data Type Conversion11/1 -> Switch30/2, Switch30/1
  Data Type Conversion7/1 -> Switch33/2, Switch33/1
  Data Type Conversion4/1 -> Switch34/2, Switch34/1
  Data Type Conversion15/1 -> Switch32/2, Switch32/1
  Data Type Conversion17/1 -> Switch35/2, Switch35/1
  LL_LFClb_TFC_KpV2_C=40/1 -> Switch35/3
  Data Type Conversion14/1 -> Switch31/2, Switch31/1
  LL_LFClb_TFC_KpVehSpdUpr_C=120/1 -> Switch34/3
  LL_LFClb_TFC_KpKlat_C=-4.5/1 -> Switch30/3
  LL_LFClb_TFC_FfCtlRatio_C=1/1 -> Switch36/3
  Data Type Conversion18/1 -> Switch36/1, Switch36/2
  Switch36/1 -> Bus Creator2/8  "LL_LFClb_TFC_FfCtlRatio_C"
  Switch40/1 -> Bus Creator2/10  "LL_LFClb_TFC_Ki_C"
  Switch39/1 -> Bus Creator2/9  "LL_LFClb_TFC_KiMaxSWA_C"
  LL_LFClb_TFC_KiMaxSWA_C=5/1 -> Switch39/3
  Data Type Conversion28/1 -> Switch39/1, Switch39/2
  LL_LFClb_TFC_Ki_C=0.01/1 -> Switch40/3
  Data Type Conversion29/1 -> Switch40/1, Switch40/2
  Data Type Conversion31/1 -> Switch42/2, Switch42/1
  LL_LKASWASyn_TrqMax=1.5/1 -> Switch42/3
  LL_LKASWASyn_SWAaddMax=8/1 -> Switch43/3
  Data Type Conversion32/1 -> Switch43/1, Switch43/2
  Switch43/1 -> Bus Creator3/1  "LL_LKASWASyn_SWAaddMax"
  Switch42/1 -> Bus Creator3/2  "LL_LKASWASyn_TrqMax"
  Bus Creator3/1 -> Bus Creator/15  "LL_LKASWAClb"
  Switch44/1 -> Bus Creator4/4  "LL_LKAExPrcs_ExitC0Dvt"
  Switch45/1 -> Bus Creator4/3  "LL_LKAExPrcs_tiExitTime3"
  Data Type Conversion34/1 -> Switch45/2, Switch45/1
  LL_LKAExPrcs_tiExitTime3=0.2/1 -> Switch45/3
  LL_LKAExPrcs_ExitC0Dvt=0.01/1 -> Switch44/3
  Data Type Conversion33/1 -> Switch44/1, Switch44/2
  Bus Creator4/1 -> Bus Creator/16  "LL_LKAExPrcs"
  Data Type Conversion35/1 -> Switch46/2, Switch46/1
  LL_LKAExPrcs_ExitC0Swt=1/1 -> Switch46/3
  Switch46/1 -> Bus Creator4/5  "LL_LKAExPrcs_ExitC0Swt"
  Switch47/1 -> Bus Creator3/3  "LL_LKASWASyn_TrqSwaAddSwt"
  LL_LKASWASyn_TrqSwaAddSwt=1/1 -> Switch47/3
  Data Type Conversion47/1 -> Switch47/1, Switch47/2
  Switch49/1 -> Bus Creator2/11  "LL_LFClb_TFC_KdMaxSWA_C"
  LL_LFClb_TFC_KdMaxSWA_C=20/1 -> Switch49/3
  Data Type Conversion49/1 -> Switch49/1, Switch49/2
  Data Type Conversion50/1 -> Switch50/2, Switch50/1
  LL_LKASWASyn_tiTrqSwaTime=0.3/1 -> Switch50/3
  Switch50/1 -> Bus Creator3/4  "LL_LKASWASyn_tiTrqSwaTime"
  Switch52/1 -> Bus Creator3/5  "LL_LKASWASyn_tiTrqSwaRtTime"
  LL_LKASWASyn_tiTrqSwaRtTime=0.2/1 -> Switch52/3
  Data Type Conversion52/1 -> Switch52/1, Switch52/2
  Data Type Conversion53/1 -> Switch53/2, Switch53/1
  LL_LKASWASyn_TrqSwaRateDiff=-0.2/1 -> Switch53/3
  Switch53/1 -> Bus Creator3/6  "LL_LKASWASyn_TrqSwaRateDiff"
  LL_LKAExPrcs_tiExitTime3=4/1 -> Switch54/3
  Data Type Conversion54/1 -> Switch54/1, Switch54/2
  Switch54/1 -> Bus Creator4/2  "LL_LKAExPrcs_tiExitTime2"
  Switch55/1 -> Bus Creator4/1  "LL_LKAExPrcs_tiExitTime1"
  Data Type Conversion55/1 -> Switch55/2, Switch55/1
  LL_LKAExPrcs_tiExitTime3=8/1 -> Switch55/3
  Switch9/1 -> Bus Creator2/16  "LL_LFClb_TFC_KdBalance_C"
  LL_LFClb_TFC_KdBalance_C=1.2/1 -> Switch9/3
  Data Type Conversion9/1 -> Switch9/1, Switch9/2
  [LLL_LKASWASyn_T2] -> Data Type Conversion24/1
  Switch16/1 -> Bus Creator3/10  "LL_LKASWASyn_T2"
  LL_LKASWASyn_T2=4/1 -> Switch16/3
  Data Type Conversion24/1 -> Switch16/1, Switch16/2
  Data Type Conversion20/1 -> Switch14/2, Switch14/1
  LL_LKASWASyn_M2=0.3/1 -> Switch14/3
  Switch14/1 -> Bus Creator3/9  "LL_LKASWASyn_M2"
  [LLL_LKASWASyn_M2] -> Data Type Conversion20/1
  [LLL_LKASWASyn_M1] -> Data Type Conversion19/1
  Switch13/1 -> Bus Creator3/8  "LL_LKASWASyn_M1"
  LL_LKASWASyn_M1=0.8/1 -> Switch13/3
  Data Type Conversion19/1 -> Switch13/1, Switch13/2
  Data Type Conversion12/1 -> Switch11/2, Switch11/1
  LL_LKASWASyn_M0=0.4/1 -> Switch11/3
  Switch11/1 -> Bus Creator3/7  "LL_LKASWASyn_M0"
  [LLL_LKASWASyn_M0] -> Data Type Conversion12/1
  Data Type Conversion25/1 -> Switch18/2, Switch18/1
  LL_LKASWASyn_M3K_DT=0.2/1 -> Switch18/3
  Switch18/1 -> Bus Creator3/11  "LL_LKASWASyn_M3K_DT"
